simulink subsystem "s_rx_uart"  (R2024b)
settings: Solver=VariableStepAuto  StartTime=0.0  StopTime=10.0  RelTol=1e-3
settings Model: Creator=marwa  LastModifiedBy=marwa

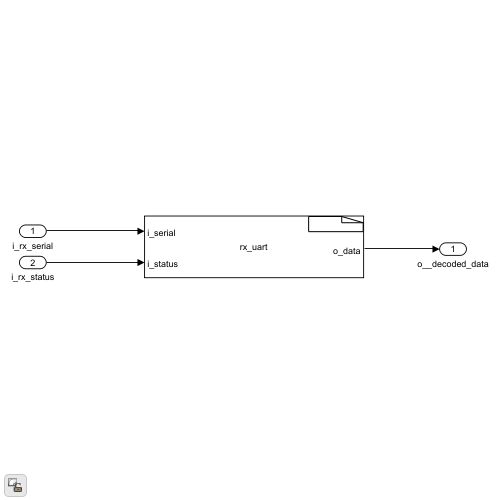
[thumbnail: Simulink's stored preview of the top-level diagram]
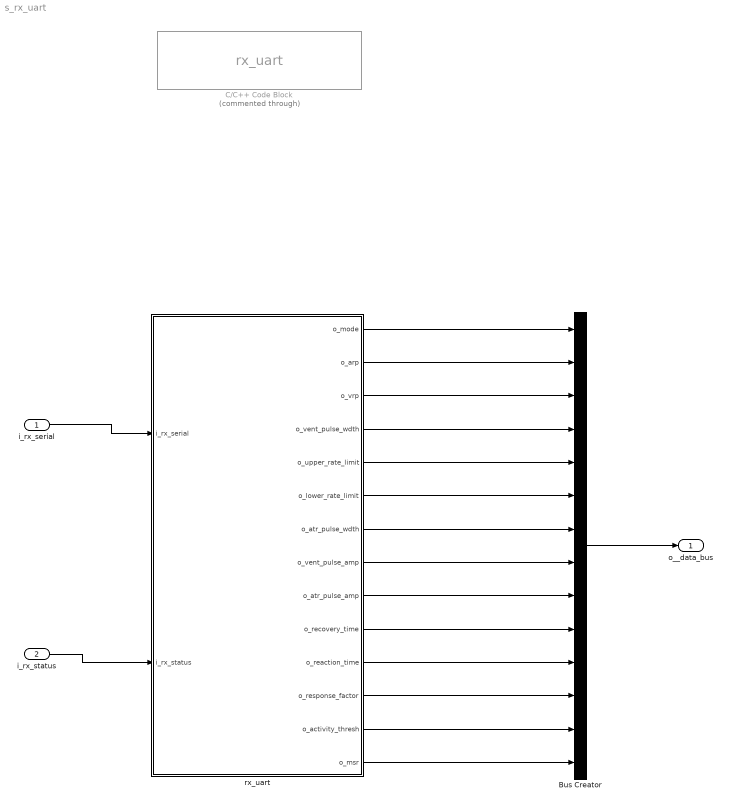
== system s_rx_uart ==
  i_rx_serial : Inport
  i_rx_status : Inport  Port=2
  Bus Creator : BusCreator  Inputs=14
  C/C++ Code Block : S-Function  Commented=through  FunctionName=rx_uart  SFunctionModules=rx_uart_wrapper.c  SFunctionDeploymentMode=off  EnableBusSupport=off  mask(S-Function Builder){}
      mask help: Simulink:masks:SFunctionBuilder_MD
      mask init:
      | val = [[.9  0.75 0.75 1 1 .9 .9 1]',[1 1 0.75 0.75 .9 .9 1 .9]'];try , sys = get_param(gcb,'SfunBuilderFcnName');if isempty(sys), sys = get_param(gcb,'FunctionName'); end,catch, sys = get_param(gcb,'FunctionName'); end
      settings: CopyFcn=set_param(gcbh,'LinkStatus','none')  OpenFcn=sfunctionwizard(gcbh)
      mask Display:
      | plot(val(:,1),val(:,2))
      | disp(sys)
      | port_label('input',1,sprintf('%s', 'i\_serial'),'interpreter','tex')
      | port_label('input',2,sprintf('%s', 'i\_status'),'interpreter','tex')
      | port_label('output',1,sprintf('%s', 'o\_data'),'interpreter','tex')
      | port_label('output',2,sprintf('%s', 'o\_new\_frame'),'interpreter','tex')
  rx_uart : Stateflow chart  TreatAsAtomicUnit=on
  o__data_bus : Outport  OutDataTypeStr=uint8
  wires:
  i_rx_serial/1 -> rx_uart/1(i_rx_serial)
  i_rx_status/1 -> rx_uart/2(i_rx_status)
  Bus Creator/1 -> o__data_bus/1
  rx_uart/1(o_mode) -> Bus Creator/1
  rx_uart/2(o_arp) -> Bus Creator/2
  rx_uart/3(o_vrp) -> Bus Creator/3
  rx_uart/4(o_vent_pulse_wdth) -> Bus Creator/4
  rx_uart/5(o_upper_rate_limit) -> Bus Creator/5
  rx_uart/6(o_lower_rate_limit) -> Bus Creator/6
  rx_uart/7(o_atr_pulse_wdth) -> Bus Creator/7
  rx_uart/9(o_atr_pulse_amp) -> Bus Creator/9
  rx_uart/8(o_vent_pulse_amp) -> Bus Creator/8
  rx_uart/10(o_recovery_time) -> Bus Creator/10
  rx_uart/11(o_reaction_time) -> Bus Creator/11
  rx_uart/12(o_response_factor) -> Bus Creator/12
  rx_uart/13(o_activity_thresh) -> Bus Creator/13
  rx_uart/14(o_msr) -> Bus Creator/14

== stateflow chart s_rx_uart/rx_uart ==
  state Initial
    entry:
    o_mode = uint8(8);
    o_lower_rate_limit = uint8(60);
    o_upper_rate_limit = uint8(120);
    o_atr_pulse_amp = uint8(3.5 / 5 * 100);
    o_atr_pulse_wdth = uint8(1);
    o_vent_pulse_amp = uint8(2.5 / 5 * 100);
    o_vent_pulse_wdth = uint8(1);
    o_arp = uint8(320);
    o_vrp = uint8(250);
    o_recovery_time = uint8(300); % in sec
    o_reaction_time = uint8(30); % in seconds
    o_response_factor = uint8(8);
    o_activity_thresh = uint8(0);
    o_msr = uint8(120);
  state Wait
  state set_params
    entry:
    o_mode = i_rx_serial(3);
    o_lower_rate_limit = i_rx_serial(4);
    o_upper_rate_limit = i_rx_serial(5);
    o_atr_pulse_amp = i_rx_serial(6);
    o_atr_pulse_wdth = i_rx_serial(7);
    o_vent_pulse_amp = i_rx_serial(8);
    o_vent_pulse_wdth = i_rx_serial(9);
    o_arp = i_rx_serial(10);
    o_vrp = i_rx_serial(11);
    o_recovery_time = i_rx_serial(12);
    o_reaction_time = i_rx_serial(13);
    o_response_factor = i_rx_serial(14);
    o_activity_thresh = i_rx_serial(15);
    o_msr = i_rx_serial(16);
  state loop_back
    entry:
    drive_outputs();
  (default) -> Initial
  Initial -> Wait
  (junction 12) -> Wait [order 2]
  Wait -> (junction 12) : [i_rx_status == 0]
  (junction 12) -> (junction 15) [order 1] : [i_rx_serial(1) == hex2dec('170')]
  (junction 15) -> set_params [order 1] : [i_rx_serial(2) == hex2dec('187')]
  (junction 15) -> loop_back [order 2] : [i_rx_serial(2) == hex2dec('204')]
  data: i_rx_serial input; i_rx_status input; o_mode output; o_arp output; o_vrp output; o_vent_pulse_wdth output; o_upper_rate_limit output; o_lower_rate_limit output; o_atr_pulse_wdth output; o_vent_pulse_amp output; o_atr_pulse_amp output; o_recovery_time output; o_reaction_time output; o_response_factor output; o_activity_thresh output; o_msr output
